simulink model "ex_anti_windup_op_PI"  (R2024a)
settings: Solver=VariableStepAuto  StartTime=0.0  StopTime=100  MaxStep=0.01  RelTol=1e-3
StopFcn:
  | figure(1);
  | 
  | subplot(211);
  | plot(r.time,r.data,y.time,y.data);
  | ylabel('r, y');
  | xlabel('Temps (s)');
  | 
  | subplot(212);
  | plot(u.time,u.data);
  | ylabel('u');
  | xlabel('Temps (s)');
settings Model: Creator=eric  LastModifiedBy=sabri
settings SolverCC: AlgebraicLoopSolver=TrustRegion
settings DataIOCC: SaveTime=off  ReturnWorkspaceOutputs=off
settings DebuggingCC: UnconnectedInputMsg=warning  UnconnectedOutputMsg=warning  UnconnectedLineMsg=warning
settings ModelReferenceCC: EnableRefExpFcnMdlSchedulingChecks=on
settings RTWCC: GPUComputeCapability=3.5

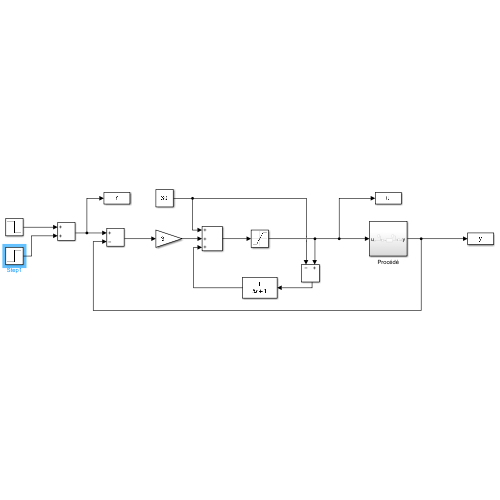
[thumbnail: Simulink's stored preview of the top-level diagram]
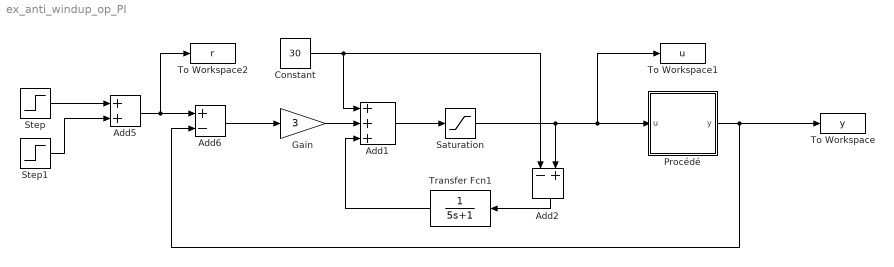
== system ex_anti_windup_op_PI ==
  Add1 : Sum  Inputs=+++
  Add2 : Sum  Inputs=-+
  Add5 : Sum
  Add6 : Sum  Inputs=+-
  Constant : Constant  Value=30
  Gain : Gain  Gain=3
  Procédé : Subsystem
  Saturation : Saturate  UpperLimit=50  LowerLimit=20
  Step : Step  Time=10  Before=40  After=30  SampleTime=0
  Step1 : Step  Time=60  After=15  SampleTime=0
  To Workspace : ToWorkspace  VariableName=y  SaveFormat=Timeseries  SampleTime=-1
  To Workspace1 : ToWorkspace  VariableName=u  SaveFormat=Timeseries  SampleTime=-1
  To Workspace2 : ToWorkspace  VariableName=r  SaveFormat=Timeseries  SampleTime=-1
  Transfer Fcn1 : TransferFcn  Denominator=[5 1]
  wires:
  Step/1 -> Add5/1
  Add6/1 -> Gain/1
  Gain/1 -> Add1/2
  Add1/1 -> Saturation/1
  Saturation/1 -> To Workspace1/1, Procédé/1(u), Add2/2
  Add2/1 -> Transfer Fcn1/1
  Constant/1 -> Add2/1, Add1/1
  Transfer Fcn1/1 -> Add1/3
  Step1/1 -> Add5/2
  Add5/1 -> To Workspace2/1, Add6/1
  Procédé/1(y) -> To Workspace/1, Add6/2

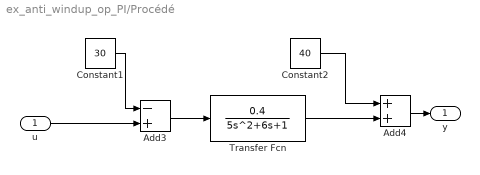
== system ex_anti_windup_op_PI/Procédé ==
  u : Inport
  Add3 : Sum  Inputs=-+
  Add4 : Sum
  Constant1 : Constant  Value=30
  Constant2 : Constant  Value=40
  Transfer Fcn : TransferFcn  Numerator=[0.4]  Denominator=[5 6 1]
  y : Outport
  wires:
  u/1 -> Add3/2
  Constant2/1 -> Add4/1
  Transfer Fcn/1 -> Add4/2
  Add4/1 -> y/1
  Constant1/1 -> Add3/1
  Add3/1 -> Transfer Fcn/1
